simulink model "Blokdiagram_100"  (R2019a)
settings: Solver=VariableStepAuto  StartTime=0.0  StopTime=28800  RelTol=1E-10
settings Model: Creator=Anton  LastModifiedBy=Anton
settings SolverCC: ZeroCrossAlgorithm=Adaptive
settings DebuggingCC: IgnoredZcDiagnostic=none

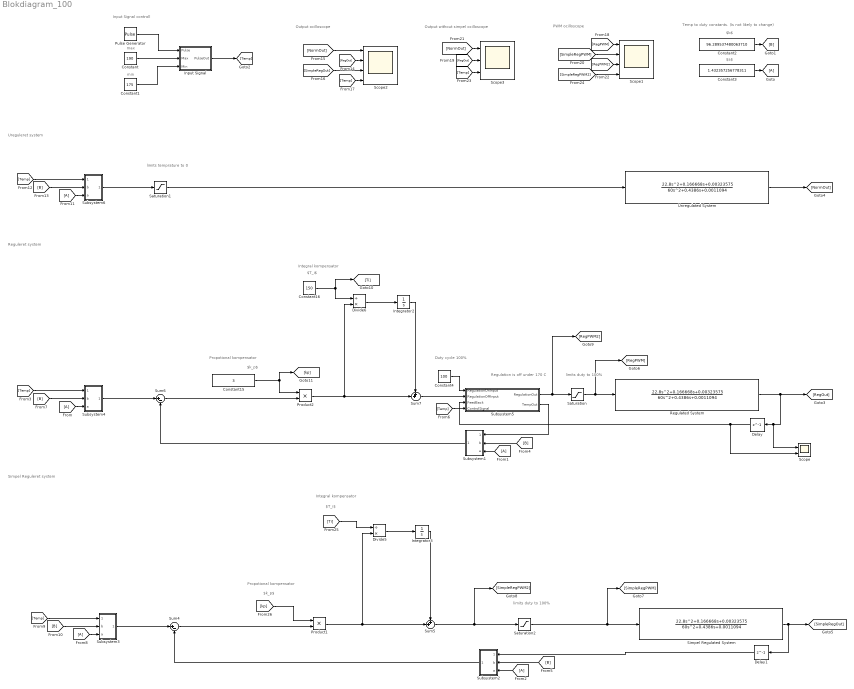
== system Blokdiagram_100 ==
  note: Reguleret system
  note: Ureguleret system
  note: Temp to duty constants. (Is not likely to change)
  note: Duty cycle
      | 100%
  note: Integral kompensator
  note: $k_p$
  note: min
  note: max
  note: $b$
  note: $a$
  note: $k_p$
  note: Propotional kompensator
  note: Propotional kompensator
  note: Integral kompensator
  note: limits
      | temprature to 0
  note: limits
      | duty to 100%
  note: Regulation is off
      | under 170 C
  note: Input Signal controll
  note: Output ocilloscope
  note: PWM ocilloscope
  note: Output without simpel ocilloscope
  note: Simpel Reguleret system
  note: $T_i$
  note: $T_i$
  note: limits
      | duty to 100%
  Constant : Constant  Value=190
  Constant1 : Constant  Value=175
  Constant15 : Constant  Value=3
  Constant16 : Constant  Value=150
  Constant2 : Constant  Value=96.289537480063710
  Constant3 : Constant  Value=1.432357256778311
  Constant4 : Constant  Value=100
  Delay : Delay  DelayLength=1  InitialCondition=0  SampleTime=0.01
  Delay1 : Delay  DelayLength=1  InitialCondition=0  SampleTime=0.01
  Divide5 : Product  Inputs=/*
  Divide6 : Product  Inputs=/*
  Input Signal : Subsystem
  Integrator2 : Integrator
  Integrator3 : Integrator
  Product1 : Product
  Product2 : Product
  Pulse Generator : DiscretePulseGenerator  PulseType=Time based  Period=14400  PulseWidth=50  PhaseDelay=7200
  Regulated System : TransferFcn  Numerator=[22.8,0.166668,0.00323575]  Denominator=[60,0.4386,0.0011094]
  Saturation : Saturate  UpperLimit=100  LowerLimit=0
  Saturation1 : Saturate  UpperLimit=400  LowerLimit=0
  Saturation2 : Saturate  UpperLimit=100  LowerLimit=0
  Scope : Scope  NumInputPorts=2
  Scope1 : Scope  NumInputPorts=4
  Scope2 : Scope  NumInputPorts=4
  Scope3 : Scope  NumInputPorts=3
  Simpel Regulated System : TransferFcn  Numerator=[22.8,0.166668,0.00323575]  Denominator=[60,0.4386,0.0011094]
  Subsystem1 : Subsystem
  Subsystem2 : Subsystem
  Subsystem3 : Subsystem
  Subsystem4 : Subsystem
  Subsystem5 : Subsystem
  Subsystem6 : Subsystem
  Sum4 : Sum  Inputs=|+-
  Sum5 : Sum  Inputs=++|
  Sum6 : Sum  Inputs=|+-
  Sum7 : Sum  Inputs=++|
  Unregulated System : TransferFcn  Numerator=[22.8,0.166668,0.00323575]  Denominator=[60,0.4386,0.0011094]
  wires:
  Simpel Regulated System/1 -> Delay1/1, [SimpleRegOut]
  Product1/1 -> Divide5/2, Sum5/2
  [kp] -> Product1/1
  Divide5/1 -> Integrator3/1
  Sum4/1 -> Product1/2
  [Ti] -> Divide5/1
  Sum5/1 -> [SimpleRegPWM2], Saturation2/1
  Product2/1 -> Divide6/2, Sum7/2
  Constant15/1 -> Product2/1, [kp]
  Regulated System/1 -> [RegOut], Scope/1, Delay/1
  Sum6/1 -> Product2/2
  Divide6/1 -> Integrator2/1
  Constant16/1 -> [Ti], Divide6/1
  Subsystem4/1(Duty) -> Sum6/1
  Pulse Generator/1 -> Input Signal/1(Pulse)
  Constant/1 -> Input Signal/2(Max)
  Constant1/1 -> Input Signal/3(Min)
  Subsystem1/1(Duty) -> Sum6/2
  Subsystem2/1(Duty) -> Sum4/2
  Saturation1/1 -> Unregulated System/1
  Constant4/1 -> Subsystem5/1(RegulationOnInput)
  Sum7/1 -> Subsystem5/2(RegulationOffInput)
  Subsystem5/1(RegulationOut) -> [RegPWM2], Saturation/1
  Subsystem5/2(TempOut) -> Subsystem1/1(Temp)
  [A] -> Subsystem4/3(a)
  Constant3/1 -> [A]
  [A] -> Subsystem1/3(a)
  [A] -> Subsystem2/3(a)
  Constant2/1 -> [B]
  [B] -> Subsystem1/2(b)
  [B] -> Subsystem2/2(b)
  [B] -> Subsystem4/2(b)
  Input Signal/1(PulseOut) -> [Temp]
  [Temp] -> Subsystem4/1(Temp)
  [Temp] -> Subsystem5/4(ControlSignal)
  [B] -> Subsystem3/2(b)
  [A] -> Subsystem3/3(a)
  [Temp] -> Subsystem3/1(Temp)
  Subsystem3/1(Duty) -> Sum4/1
  [B] -> Subsystem6/2(b)
  [A] -> Subsystem6/3(a)
  [Temp] -> Subsystem6/1(Temp)
  [RegOut] -> Scope2/2
  Unregulated System/1 -> [NormOut]
  [NormOut] -> Scope2/1
  [SimpleRegOut] -> Scope2/3
  [Temp] -> Scope2/4
  [SimpleRegPWM] -> Scope1/2
  [RegPWM] -> Scope1/1
  [Temp] -> Scope3/3
  [RegOut] -> Scope3/2
  [NormOut] -> Scope3/1
  Saturation/1 -> Regulated System/1, [RegPWM]
  Saturation2/1 -> [SimpleRegPWM], Simpel Regulated System/1
  [SimpleRegPWM2] -> Scope1/4
  [RegPWM2] -> Scope1/3
  Subsystem6/1(Duty) -> Saturation1/1
  Integrator2/1 -> Sum7/1
  Integrator3/1 -> Sum5/1
  Delay/1 -> Scope/2, Subsystem5/3(FeedBack)
  Delay1/1 -> Subsystem2/1(Temp)

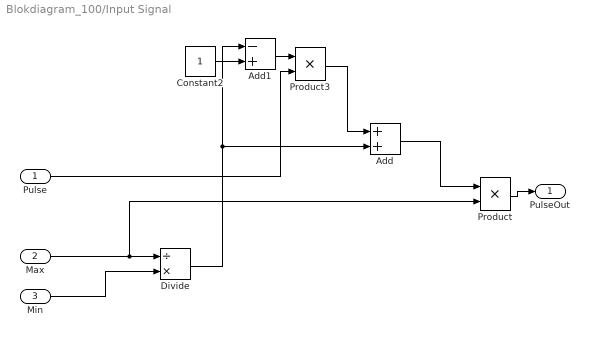
== system Blokdiagram_100/Input Signal ==
  Pulse : Inport
  Max : Inport  Port=2
  Min : Inport  Port=3
  Add : Sum
  Add1 : Sum  Inputs=-+
  Constant2 : Constant
  Divide : Product  Inputs=/*
  Product : Product
  Product3 : Product
  PulseOut : Outport
  wires:
  Constant2/1 -> Add1/2
  Divide/1 -> Add/2, Add1/1
  Product3/1 -> Add/1
  Max/1 -> Product/2, Divide/1
  Add1/1 -> Product3/1
  Pulse/1 -> Product3/2
  Add/1 -> Product/1
  Min/1 -> Divide/2
  Product/1 -> PulseOut/1

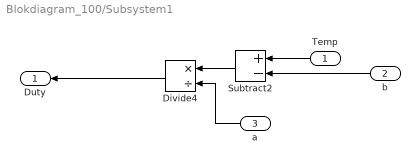
== system Blokdiagram_100/Subsystem1 ==
  Temp : Inport
  b : Inport  Port=2
  a : Inport  Port=3
  Divide4 : Product  Inputs=*/
  Subtract2 : Sum  Inputs=+-
  Duty : Outport
  wires:
  a/1 -> Divide4/2
  Divide4/1 -> Duty/1
  Subtract2/1 -> Divide4/1
  Temp/1 -> Subtract2/1
  b/1 -> Subtract2/2

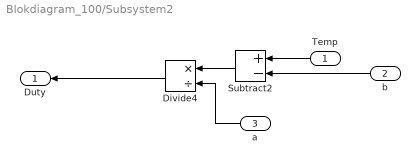
== system Blokdiagram_100/Subsystem2 ==
  Temp : Inport
  b : Inport  Port=2
  a : Inport  Port=3
  Divide4 : Product  Inputs=*/
  Subtract2 : Sum  Inputs=+-
  Duty : Outport
  wires:
  a/1 -> Divide4/2
  Divide4/1 -> Duty/1
  Subtract2/1 -> Divide4/1
  Temp/1 -> Subtract2/1
  b/1 -> Subtract2/2

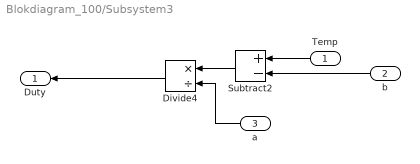
== system Blokdiagram_100/Subsystem3 ==
  Temp : Inport
  b : Inport  Port=2
  a : Inport  Port=3
  Divide4 : Product  Inputs=*/
  Subtract2 : Sum  Inputs=+-
  Duty : Outport
  wires:
  a/1 -> Divide4/2
  Divide4/1 -> Duty/1
  Subtract2/1 -> Divide4/1
  Temp/1 -> Subtract2/1
  b/1 -> Subtract2/2

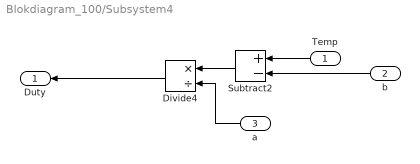
== system Blokdiagram_100/Subsystem4 ==
  Temp : Inport
  b : Inport  Port=2
  a : Inport  Port=3
  Divide4 : Product  Inputs=*/
  Subtract2 : Sum  Inputs=+-
  Duty : Outport
  wires:
  a/1 -> Divide4/2
  Divide4/1 -> Duty/1
  Subtract2/1 -> Divide4/1
  Temp/1 -> Subtract2/1
  b/1 -> Subtract2/2

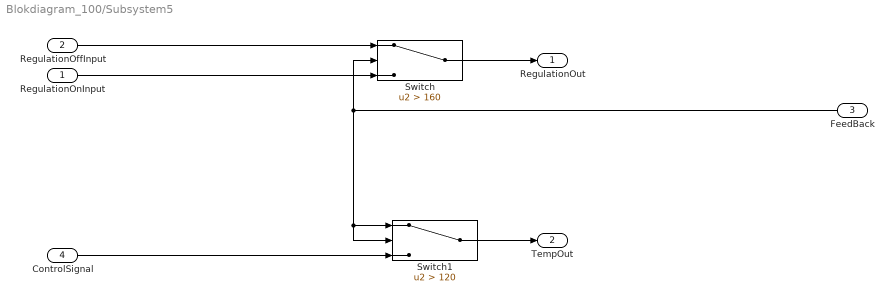
== system Blokdiagram_100/Subsystem5 ==
  RegulationOnInput : Inport
  RegulationOffInput : Inport  Port=2
  FeedBack : Inport  Port=3
  ControlSignal : Inport  Port=4
  Switch : Switch  Criteria=u2 > Threshold  Threshold=160
  Switch1 : Switch  Criteria=u2 > Threshold  Threshold=120
  RegulationOut : Outport
  TempOut : Outport  Port=2
  wires:
  ControlSignal/1 -> Switch1/3
  FeedBack/1 -> Switch/2, Switch1/1, Switch1/2
  Switch1/1 -> TempOut/1
  RegulationOffInput/1 -> Switch/1
  Switch/1 -> RegulationOut/1
  RegulationOnInput/1 -> Switch/3

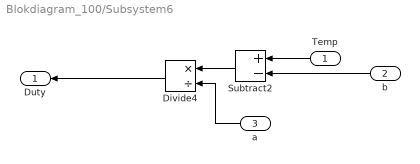
== system Blokdiagram_100/Subsystem6 ==
  Temp : Inport
  b : Inport  Port=2
  a : Inport  Port=3
  Divide4 : Product  Inputs=*/
  Subtract2 : Sum  Inputs=+-
  Duty : Outport
  wires:
  a/1 -> Divide4/2
  Divide4/1 -> Duty/1
  Subtract2/1 -> Divide4/1
  Temp/1 -> Subtract2/1
  b/1 -> Subtract2/2
